simulink model "LAB3_BPSK_Mod_Demod"  (R2020a)
settings: Solver=VariableStepAuto  StartTime=0.0  StopTime=10.0  RelTol=1e-3
libraries: dspsigops x3, simulink_extras x2, simulink x1, dspsrcs4 x1
settings Model: Creator=Sameer  LastModifiedBy=Sameer

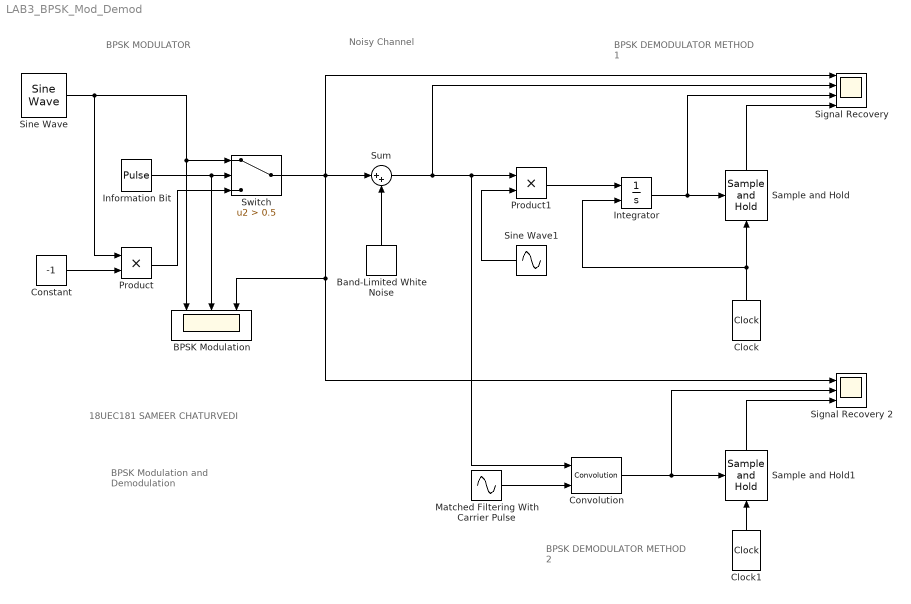
== system LAB3_BPSK_Mod_Demod ==
  note: Noisy Channel
  note: BPSK Modulation
      | and Demodulation
  note: BPSK MODULATOR
  note: 18UEC181
      | SAMEER CHATURVEDI
  note: BPSK DEMODULATOR
      | METHOD 1
  note: BPSK DEMODULATOR
      | METHOD 2
  BPSK Modulation : Scope  NumInputPorts=3
  Band-Limited White Noise : simulink/Sources/Band-Limited White Noise  Cov=[0.005]  Ts=0.1  seed=[23341]
  Clock : simulink_extras/Flip Flops/Clock  period=2
  Clock1 : simulink_extras/Flip Flops/Clock  period=2
  Constant : Constant  Value=-1
  Convolution : dspsigops/Convolution  domain=Time  roundingMode=Floor  overflowMode=off  outputDataTypeStr=Inherit: Same as accumulator  outputMin=[]  outputMax=[]  outputLastDataTypeStr=Inherit: Same as accumulator
      settings: SourceProductBaseCode=DS
  Information Bit : DiscretePulseGenerator  PulseType=Time based  PulseWidth=50
  Integrator : Integrator  ExternalReset=either
  Matched Filtering With Carrier Pulse : Sin  Frequency=2*pi*2  SampleTime=0.001
  Product : Product
  Product1 : Product
  Sample and Hold : dspsigops/Sample and Hold  trig=Rising edge  initCond=0  latchinput=off
  Sample and Hold1 : dspsigops/Sample and Hold  trig=Either edge  initCond=0  latchinput=off
  Signal Recovery : Scope  NumInputPorts=4
  Signal Recovery 2 : Scope  NumInputPorts=3
  Sine Wave : dspsrcs4/Sine Wave  Amplitude=1  Frequency=2  Phase=0  SampleMode=Discrete  OutComplex=Real  CompMethod=Trigonometric fcn  TableSize=Speed  SampleTime=1/1000  SamplesPerFrame=1  ResetState=Restart at time zero  OutputFrames=off  dataType=double  wordLen=16  udDataType=sfix(16)  fracBitsMode=Best precision  numFracBits=15  OutDataTypeStr=double  LastOutDataTypeStr=double
  Sine Wave1 : Sin  Frequency=2*pi*2  SampleTime=0.001
  Sum : Sum  Inputs=|++
  Switch : Switch  Criteria=u2 > Threshold  Threshold=0.5
  wires:
  Constant/1 -> Product/2
  Product/1 -> Switch/3
  Switch/1 -> Signal Recovery/1, BPSK Modulation/3, Signal Recovery 2/1, Sum/1
  Information Bit/1 -> Switch/2, BPSK Modulation/2
  Sine Wave/1 -> Product/1, Switch/1, BPSK Modulation/1
  Band-Limited White Noise/1 -> Sum/2
  Sine Wave1/1 -> Product1/2
  Sum/1 -> Signal Recovery/2, Product1/1, Convolution/1
  Product1/1 -> Integrator/1
  Integrator/1 -> Signal Recovery/3, Sample and Hold/Trigger
  Clock/1 -> Integrator/2, Sample and Hold/1
  Sample and Hold/1 -> Signal Recovery/4
  Matched Filtering With Carrier Pulse/1 -> Convolution/2
  Convolution/1 -> Signal Recovery 2/2, Sample and Hold1/Trigger
  Clock1/1 -> Sample and Hold1/1
  Sample and Hold1/1 -> Signal Recovery 2/3
